simulink library "inp"  (R2021b)
settings: Solver=VariableStepAuto  StartTime=0.0  StopTime=10.0  RelTol=1e-3
undefined symbols (not defined in the file): C_TASK_5MS_S, FALSE, KINP_AcoreReadyToSlp_flg_ovrdflg, KINP_AcoreReadyToSlp_flg_ovrdval, KINP_AllowMovThd_OTA_enum_ovrdflg, KINP_AllowMovThd_OTA_enum_ovrdval, KINP_APSAngleTarget_Deg_ovrdflg, KINP_APSAngleTarget_Deg_ovrdval, KINP_APSDecReq_mps2_ovrdflg, KINP_APSDecReq_mps2_ovrdval, KINP_APSDecReqA_flg_ovrdflg, KINP_APSDecReqA_flg_ovrdval, KINP_APSDFLL_cm_ovrdflg, KINP_APSDFLL_cm_ovrdval, KINP_APSDFLR_cm_ovrdflg, KINP_APSDFLR_cm_ovrdval, KINP_APSDRLL_cm_ovrdflg, KINP_APSDRLL_cm_ovrdval, KINP_APSDRLR_cm_ovrdflg, KINP_APSDRLR_cm_ovrdval, KINP_APSExitCondition_enum_ovrdflg, KINP_APSExitCondition_enum_ovrdval, KINP_APSHWVer_enum_ovrdflg, KINP_APSHWVer_enum_ovrdval, KINP_APSProgressPCT_pct_ovrdflg, KINP_APSProgressPCT_pct_ovrdval, KINP_APSPwrReq_enum_ovrdflg, KINP_APSPwrReq_enum_ovrdval, KINP_APSReq_enum_ovrdflg, KINP_APSReq_enum_ovrdval, KINP_APSRQDisplay_enum_ovrdflg, KINP_APSRQDisplay_enum_ovrdval, KINP_APSRqEPASCtrl_flg_ovrdflg, KINP_APSRqEPASCtrl_flg_ovrdval, KINP_APSShiftPosnReq_enum_ovrdval, KINP_APSShiftPosnReq_enum_ovrflg, KINP_APSSpeedCMD_kph_ovrdval, KINP_APSSpeedCMD_kph_ovrflg, KINP_APSStaSystem_enum_ovrdflg, KINP_APSStaSystem_enum_ovrdval, KINP_APSSWVer_enum_ovrdflg, KINP_APSSWVer_enum_ovrdval, KINP_APSVMCReqA_flg_ovrdval, KINP_APSVMCReqA_flg_ovrflg, KINP_APSVRqEPASCtrl_flg_ovrdflg, KINP_APSVRqEPASCtrl_flg_ovrdval, KINP_AuxBattVolmV_mV_ovrdflg, KINP_AuxBattVolmV_mV_ovrdval, KINP_BTConnectSta_enum_ovrdflg, KINP_BTConnectSta_enum_ovrdval, KINP_CAASSta_enum_ovrdflg, KINP_CAASSta_enum_ovrdval, KINP_CAASVMCReqA_flg_ovrdval, KINP_CAASVMCReqA_flg_ovrflg, KINP_CAN1BusOff_flg_ovrdflg, KINP_CAN1BusOff_flg_ovrdval, KINP_CAN2BusOff_flg_ovrdflg, KINP_CAN2BusOff_flg_ovrdval, KINP_CAN3BusOff_flg_ovrdflg, KINP_CAN3BusOff_flg_ovrdval ... (+222)
libraries: FVT_lib x1035, hcu_lib x1
(part 14 of 33)

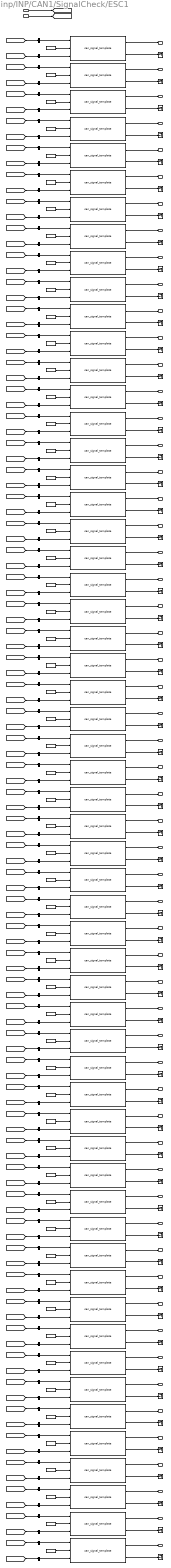
== system inp/INP/CAN1/SignalCheck/ESC1 ==
  BHAL_outputs : Inport
  inp_CanValid_bus : Inport  Port=2
  ABSActive : FVT_lib/inp/can_signal_template  SystemSampleTime=-1  VariantActivationTime=update diagram  Latency=0  AutoFrameSizeCalculation=off
      link override defval: Value=KINP_ABSActive_flg_defval
      link override ovrdflg: Value=KINP_ABSActive_flg_ovrdflg
      link override ovrdval: Value=KINP_ABSActive_flg_ovrdval
  ABSFailed : FVT_lib/inp/can_signal_template  SystemSampleTime=-1  VariantActivationTime=update diagram  Latency=0  AutoFrameSizeCalculation=off
      link override defval: Value=KINP_ABSFailed_flg_defval
      link override ovrdflg: Value=KINP_ABSFailed_flg_ovrdflg
      link override ovrdval: Value=KINP_ABSFailed_flg_ovrdval
  ABSWnlmpSta : FVT_lib/inp/can_signal_template  SystemSampleTime=-1  VariantActivationTime=update diagram  Latency=0  AutoFrameSizeCalculation=off
      link override defval: Value=KINP_ABSWnlmpSta_flg_defval
      link override ovrdflg: Value=KINP_ABSWnlmpSta_flg_ovrdflg
      link override ovrdval: Value=KINP_ABSWnlmpSta_flg_ovrdval
  AVHActive : FVT_lib/inp/can_signal_template  SystemSampleTime=-1  VariantActivationTime=update diagram  Latency=0  AutoFrameSizeCalculation=off
      link override defval: Value=KINP_AVHActive_flg_defval
      link override ovrdflg: Value=KINP_AVHActive_flg_ovrdflg
      link override ovrdval: Value=KINP_AVHActive_flg_ovrdval
  AVHFailed : FVT_lib/inp/can_signal_template  SystemSampleTime=-1  VariantActivationTime=update diagram  Latency=0  AutoFrameSizeCalculation=off
      link override defval: Value=KINP_AVHFailed_flg_defval
      link override ovrdflg: Value=KINP_AVHFailed_flg_ovrdflg
      link override ovrdval: Value=KINP_AVHFailed_flg_ovrdval
  AmberWnlmpSta : FVT_lib/inp/can_signal_template  SystemSampleTime=-1  VariantActivationTime=update diagram  Latency=0  AutoFrameSizeCalculation=off
      link override defval: Value=KINP_AmberWnlmpSta_flg_defval
      link override ovrdflg: Value=KINP_AmberWnlmpSta_flg_ovrdflg
      link override ovrdval: Value=KINP_AmberWnlmpSta_flg_ovrdval
  BTCSActive : FVT_lib/inp/can_signal_template  SystemSampleTime=-1  VariantActivationTime=update diagram  Latency=0  AutoFrameSizeCalculation=off
      link override defval: Value=KINP_BTCSActive_flg_defval
      link override ovrdflg: Value=KINP_BTCSActive_flg_ovrdflg
      link override ovrdval: Value=KINP_BTCSActive_flg_ovrdval
  EBDActive : FVT_lib/inp/can_signal_template  SystemSampleTime=-1  VariantActivationTime=update diagram  Latency=0  AutoFrameSizeCalculation=off
      link override defval: Value=KINP_EBDActive_flg_defval
      link override ovrdflg: Value=KINP_EBDActive_flg_ovrdflg
      link override ovrdval: Value=KINP_EBDActive_flg_ovrdval
  EBDFailed : FVT_lib/inp/can_signal_template  SystemSampleTime=-1  VariantActivationTime=update diagram  Latency=0  AutoFrameSizeCalculation=off
      link override defval: Value=KINP_EBDFailed_flg_defval
      link override ovrdflg: Value=KINP_EBDFailed_flg_ovrdflg
      link override ovrdval: Value=KINP_EBDFailed_flg_ovrdval
  ESC1CS : FVT_lib/inp/can_signal_template  SystemSampleTime=-1  VariantActivationTime=update diagram  Latency=0  AutoFrameSizeCalculation=off
      link override defval: Value=KINP_ESC1CS_enum_defval
      link override ovrdflg: Value=KINP_ESC1CS_enum_ovrdflg
      link override ovrdval: Value=KINP_ESC1CS_enum_ovrdval
  ESC1CSErr : FVT_lib/inp/can_signal_template  SystemSampleTime=-1  VariantActivationTime=update diagram  Latency=0  AutoFrameSizeCalculation=off
      link override defval: Value=KINP_ESC1CSErr_flg_defval
      link override ovrdflg: Value=KINP_ESC1CSErr_flg_ovrdflg
      link override ovrdval: Value=KINP_ESC1CSErr_flg_ovrdval
  ESC1RC : FVT_lib/inp/can_signal_template  SystemSampleTime=-1  VariantActivationTime=update diagram  Latency=0  AutoFrameSizeCalculation=off
      link override defval: Value=KINP_ESC1RC_enum_defval
      link override ovrdflg: Value=KINP_ESC1RC_enum_ovrdflg
      link override ovrdval: Value=KINP_ESC1RC_enum_ovrdval
  ESC1RCErr : FVT_lib/inp/can_signal_template  SystemSampleTime=-1  VariantActivationTime=update diagram  Latency=0  AutoFrameSizeCalculation=off
      link override defval: Value=KINP_ESC1RCErr_flg_defval
      link override ovrdflg: Value=KINP_ESC1RCErr_flg_ovrdflg
      link override ovrdval: Value=KINP_ESC1RCErr_flg_ovrdval
  ESCActive : FVT_lib/inp/can_signal_template  SystemSampleTime=-1  VariantActivationTime=update diagram  Latency=0  AutoFrameSizeCalculation=off
      link override defval: Value=KINP_ESCActive_flg_defval
      link override ovrdflg: Value=KINP_ESCActive_flg_ovrdflg
      link override ovrdval: Value=KINP_ESCActive_flg_ovrdval
  ESCBeepReq : FVT_lib/inp/can_signal_template  SystemSampleTime=-1  VariantActivationTime=update diagram  Latency=0  AutoFrameSizeCalculation=off
      link override defval: Value=KINP_ESCBeepReq_flg_defval
      link override ovrdflg: Value=KINP_ESCBeepReq_flg_ovrdflg
      link override ovrdval: Value=KINP_ESCBeepReq_flg_ovrdval
  ESCFailed : FVT_lib/inp/can_signal_template  SystemSampleTime=-1  VariantActivationTime=update diagram  Latency=0  AutoFrameSizeCalculation=off
      link override defval: Value=KINP_ESCFailed_flg_defval
      link override ovrdflg: Value=KINP_ESCFailed_flg_ovrdflg
      link override ovrdval: Value=KINP_ESCFailed_flg_ovrdval
  ESCOFFStatus : FVT_lib/inp/can_signal_template  SystemSampleTime=-1  VariantActivationTime=update diagram  Latency=0  AutoFrameSizeCalculation=off
      link override defval: Value=KINP_ESCOFFStatus_enum_defval
      link override ovrdflg: Value=KINP_ESCOFFStatus_enum_ovrdflg
      link override ovrdval: Value=KINP_ESCOFFStatus_enum_ovrdval
  ESCOfflmpSta : FVT_lib/inp/can_signal_template  SystemSampleTime=-1  VariantActivationTime=update diagram  Latency=0  AutoFrameSizeCalculation=off
      link override defval: Value=KINP_ESCOfflmpSta_flg_defval
      link override ovrdflg: Value=KINP_ESCOfflmpSta_flg_ovrdflg
      link override ovrdval: Value=KINP_ESCOfflmpSta_flg_ovrdval
  ESCWnlmpSta : FVT_lib/inp/can_signal_template  SystemSampleTime=-1  VariantActivationTime=update diagram  Latency=0  AutoFrameSizeCalculation=off
      link override defval: Value=KINP_ESCWnlmpSta_enum_defval
      link override ovrdflg: Value=KINP_ESCWnlmpSta_enum_ovrdflg
      link override ovrdval: Value=KINP_ESCWnlmpSta_enum_ovrdval
  ESSActive : FVT_lib/inp/can_signal_template  SystemSampleTime=-1  VariantActivationTime=update diagram  Latency=0  AutoFrameSizeCalculation=off
      link override defval: Value=KINP_ESSActive_flg_defval
      link override ovrdflg: Value=KINP_ESSActive_flg_ovrdflg
      link override ovrdval: Value=KINP_ESSActive_flg_ovrdval
  FrPTCSActive : FVT_lib/inp/can_signal_template  SystemSampleTime=-1  VariantActivationTime=update diagram  Latency=0  AutoFrameSizeCalculation=off
      link override defval: Value=KINP_FrPTCSActive_flg_defval
      link override ovrdflg: Value=KINP_FrPTCSActive_flg_ovrdflg
      link override ovrdval: Value=KINP_FrPTCSActive_flg_ovrdval
  FrntAxlTrqReqDrv : FVT_lib/inp/can_signal_template  SystemSampleTime=-1  VariantActivationTime=update diagram  Latency=0  AutoFrameSizeCalculation=off
      link override defval: Value=KINP_FrntAxlTrqReqDrv_Nm_defval
      link override ovrdflg: Value=KINP_FrntAxlTrqReqDrv_Nm_ovrdflg
      link override ovrdval: Value=KINP_FrntAxlTrqReqDrv_Nm_ovrdval
  GRADE : FVT_lib/inp/can_signal_template  SystemSampleTime=-1  VariantActivationTime=update diagram  Latency=0  AutoFrameSizeCalculation=off
      link override defval: Value=KINP_GRADE_Deg_defval
      link override ovrdflg: Value=KINP_GRADE_Deg_ovrdflg
      link override ovrdval: Value=KINP_GRADE_Deg_ovrdval
  HBBActive : FVT_lib/inp/can_signal_template  SystemSampleTime=-1  VariantActivationTime=update diagram  Latency=0  AutoFrameSizeCalculation=off
      link override defval: Value=KINP_HBBActive_flg_defval
      link override ovrdflg: Value=KINP_HBBActive_flg_ovrdflg
      link override ovrdval: Value=KINP_HBBActive_flg_ovrdval
  HBBFailed : FVT_lib/inp/can_signal_template  SystemSampleTime=-1  VariantActivationTime=update diagram  Latency=0  AutoFrameSizeCalculation=off
      link override defval: Value=KINP_HBBFailed_flg_defval
      link override ovrdflg: Value=KINP_HBBFailed_flg_ovrdflg
      link override ovrdval: Value=KINP_HBBFailed_flg_ovrdval
  HDDActive : FVT_lib/inp/can_signal_template  SystemSampleTime=-1  VariantActivationTime=update diagram  Latency=0  AutoFrameSizeCalculation=off
      link override defval: Value=KINP_HDDActive_flg_defval
      link override ovrdflg: Value=KINP_HDDActive_flg_ovrdflg
      link override ovrdval: Value=KINP_HDDActive_flg_ovrdval
  HDDFailed : FVT_lib/inp/can_signal_template  SystemSampleTime=-1  VariantActivationTime=update diagram  Latency=0  AutoFrameSizeCalculation=off
      link override defval: Value=KINP_HDDFailed_flg_defval
      link override ovrdflg: Value=KINP_HDDFailed_flg_ovrdflg
      link override ovrdval: Value=KINP_HDDFailed_flg_ovrdval
  HSAActive : FVT_lib/inp/can_signal_template  SystemSampleTime=-1  VariantActivationTime=update diagram  Latency=0  AutoFrameSizeCalculation=off
      link override defval: Value=KINP_HSAActive_flg_defval
      link override ovrdflg: Value=KINP_HSAActive_flg_ovrdflg
      link override ovrdval: Value=KINP_HSAActive_flg_ovrdval
  HSAFailed : FVT_lib/inp/can_signal_template  SystemSampleTime=-1  VariantActivationTime=update diagram  Latency=0  AutoFrameSizeCalculation=off
      link override defval: Value=KINP_HSAFailed_flg_defval
      link override ovrdflg: Value=KINP_HSAFailed_flg_ovrdflg
      link override ovrdval: Value=KINP_HSAFailed_flg_ovrdval
  LFPulseCount : FVT_lib/inp/can_signal_template  SystemSampleTime=-1  VariantActivationTime=update diagram  Latency=0  AutoFrameSizeCalculation=off
      link override defval: Value=KINP_LFPulseCount_enum_defval
      link override ovrdflg: Value=KINP_LFPulseCount_enum_ovrdflg
      link override ovrdval: Value=KINP_LFPulseCount_enum_ovrdval
  LFPulseCountV : FVT_lib/inp/can_signal_template  SystemSampleTime=-1  VariantActivationTime=update diagram  Latency=0  AutoFrameSizeCalculation=off
      link override defval: Value=KINP_LFPulseCountV_flg_defval
      link override ovrdflg: Value=KINP_LFPulseCountV_flg_ovrdflg
      link override ovrdval: Value=KINP_LFPulseCountV_flg_ovrdval
  LFRawWhlSpeed : FVT_lib/inp/can_signal_template  SystemSampleTime=-1  VariantActivationTime=update diagram  Latency=0  AutoFrameSizeCalculation=off
      link override defval: Value=KINP_LFRawWhlSpeed_kph_defval
      link override ovrdflg: Value=KINP_LFRawWhlSpeed_kph_ovrdflg
      link override ovrdval: Value=KINP_LFRawWhlSpeed_kph_ovrdval
  LFRawWhlSpeedV : FVT_lib/inp/can_signal_template  SystemSampleTime=-1  VariantActivationTime=update diagram  Latency=0  AutoFrameSizeCalculation=off
      link override defval: Value=KINP_LFRawWhlSpeedV_flg_defval
      link override ovrdflg: Value=KINP_LFRawWhlSpeedV_flg_ovrdflg
      link override ovrdval: Value=KINP_LFRawWhlSpeedV_flg_ovrdval
  LFWhlRotDir : FVT_lib/inp/can_signal_template  SystemSampleTime=-1  VariantActivationTime=update diagram  Latency=0  AutoFrameSizeCalculation=off
      link override defval: Value=KINP_LFWhlRotDir_enum_defval
      link override ovrdflg: Value=KINP_LFWhlRotDir_enum_ovrdflg
      link override ovrdval: Value=KINP_LFWhlRotDir_enum_ovrdval
  LRPulseCount : FVT_lib/inp/can_signal_template  SystemSampleTime=-1  VariantActivationTime=update diagram  Latency=0  AutoFrameSizeCalculation=off
      link override defval: Value=KINP_LRPulseCount_enum_defval
      link override ovrdflg: Value=KINP_LRPulseCount_enum_ovrdflg
      link override ovrdval: Value=KINP_LRPulseCount_enum_ovrdval
  LRPulseCountV : FVT_lib/inp/can_signal_template  SystemSampleTime=-1  VariantActivationTime=update diagram  Latency=0  AutoFrameSizeCalculation=off
      link override defval: Value=KINP_LRPulseCountV_flg_defval
      link override ovrdflg: Value=KINP_LRPulseCountV_flg_ovrdflg
      link override ovrdval: Value=KINP_LRPulseCountV_flg_ovrdval
  LRRawWhlSpeed : FVT_lib/inp/can_signal_template  SystemSampleTime=-1  VariantActivationTime=update diagram  Latency=0  AutoFrameSizeCalculation=off
      link override defval: Value=KINP_LRRawWhlSpeed_kph_defval
      link override ovrdflg: Value=KINP_LRRawWhlSpeed_kph_ovrdflg
      link override ovrdval: Value=KINP_LRRawWhlSpeed_kph_ovrdval
  LRRawWhlSpeedV : FVT_lib/inp/can_signal_template  SystemSampleTime=-1  VariantActivationTime=update diagram  Latency=0  AutoFrameSizeCalculation=off
      link override defval: Value=KINP_LRRawWhlSpeedV_flg_defval
      link override ovrdflg: Value=KINP_LRRawWhlSpeedV_flg_ovrdflg
      link override ovrdval: Value=KINP_LRRawWhlSpeedV_flg_ovrdval
  LRWhlRotDir : FVT_lib/inp/can_signal_template  SystemSampleTime=-1  VariantActivationTime=update diagram  Latency=0  AutoFrameSizeCalculation=off
      link override defval: Value=KINP_LRWhlRotDir_enum_defval
      link override ovrdflg: Value=KINP_LRWhlRotDir_enum_ovrdflg
      link override ovrdval: Value=KINP_LRWhlRotDir_enum_ovrdval
  PBAActive : FVT_lib/inp/can_signal_template  SystemSampleTime=-1  VariantActivationTime=update diagram  Latency=0  AutoFrameSizeCalculation=off
      link override defval: Value=KINP_PBAActive_flg_defval
      link override ovrdflg: Value=KINP_PBAActive_flg_ovrdflg
      link override ovrdval: Value=KINP_PBAActive_flg_ovrdval
  PBAFailed : FVT_lib/inp/can_signal_template  SystemSampleTime=-1  VariantActivationTime=update diagram  Latency=0  AutoFrameSizeCalculation=off
      link override defval: Value=KINP_PBAFailed_flg_defval
      link override ovrdflg: Value=KINP_PBAFailed_flg_ovrdflg
      link override ovrdval: Value=KINP_PBAFailed_flg_ovrdval
  RFPulseCount : FVT_lib/inp/can_signal_template  SystemSampleTime=-1  VariantActivationTime=update diagram  Latency=0  AutoFrameSizeCalculation=off
      link override defval: Value=KINP_RFPulseCount_enum_defval
      link override ovrdflg: Value=KINP_RFPulseCount_enum_ovrdflg
      link override ovrdval: Value=KINP_RFPulseCount_enum_ovrdval
  RFPulseCountV : FVT_lib/inp/can_signal_template  SystemSampleTime=-1  VariantActivationTime=update diagram  Latency=0  AutoFrameSizeCalculation=off
      link override defval: Value=KINP_RFPulseCountV_flg_defval
      link override ovrdflg: Value=KINP_RFPulseCountV_flg_ovrdflg
      link override ovrdval: Value=KINP_RFPulseCountV_flg_ovrdval
  RFRawWhlSpeed : FVT_lib/inp/can_signal_template  SystemSampleTime=-1  VariantActivationTime=update diagram  Latency=0  AutoFrameSizeCalculation=off
      link override defval: Value=KINP_RFRawWhlSpeed_kph_defval
      link override ovrdflg: Value=KINP_RFRawWhlSpeed_kph_ovrdflg
      link override ovrdval: Value=KINP_RFRawWhlSpeed_kph_ovrdval
  RFRawWhlSpeedV : FVT_lib/inp/can_signal_template  SystemSampleTime=-1  VariantActivationTime=update diagram  Latency=0  AutoFrameSizeCalculation=off
      link override defval: Value=KINP_RFRawWhlSpeedV_flg_defval
      link override ovrdflg: Value=KINP_RFRawWhlSpeedV_flg_ovrdflg
      link override ovrdval: Value=KINP_RFRawWhlSpeedV_flg_ovrdval
  RFWhlRotDir : FVT_lib/inp/can_signal_template  SystemSampleTime=-1  VariantActivationTime=update diagram  Latency=0  AutoFrameSizeCalculation=off
      link override defval: Value=KINP_RFWhlRotDir_enum_defval
      link override ovrdflg: Value=KINP_RFWhlRotDir_enum_ovrdflg
      link override ovrdval: Value=KINP_RFWhlRotDir_enum_ovrdval
  RRPulseCount : FVT_lib/inp/can_signal_template  SystemSampleTime=-1  VariantActivationTime=update diagram  Latency=0  AutoFrameSizeCalculation=off
      link override defval: Value=KINP_RRPulseCount_enum_defval
      link override ovrdflg: Value=KINP_RRPulseCount_enum_ovrdflg
      link override ovrdval: Value=KINP_RRPulseCount_enum_ovrdval
  RRPulseCountV : FVT_lib/inp/can_signal_template  SystemSampleTime=-1  VariantActivationTime=update diagram  Latency=0  AutoFrameSizeCalculation=off
      link override defval: Value=KINP_RRPulseCountV_flg_defval
      link override ovrdflg: Value=KINP_RRPulseCountV_flg_ovrdflg
      link override ovrdval: Value=KINP_RRPulseCountV_flg_ovrdval
  RRRawWhlSpeed : FVT_lib/inp/can_signal_template  SystemSampleTime=-1  VariantActivationTime=update diagram  Latency=0  AutoFrameSizeCalculation=off
      link override defval: Value=KINP_RRRawWhlSpeed_kph_defval
      link override ovrdflg: Value=KINP_RRRawWhlSpeed_kph_ovrdflg
      link override ovrdval: Value=KINP_RRRawWhlSpeed_kph_ovrdval
  RRRawWhlSpeedV : FVT_lib/inp/can_signal_template  SystemSampleTime=-1  VariantActivationTime=update diagram  Latency=0  AutoFrameSizeCalculation=off
      link override defval: Value=KINP_RRRawWhlSpeedV_flg_defval
      link override ovrdflg: Value=KINP_RRRawWhlSpeedV_flg_ovrdflg
      link override ovrdval: Value=KINP_RRRawWhlSpeedV_flg_ovrdval
  RRWhlRotDir : FVT_lib/inp/can_signal_template  SystemSampleTime=-1  VariantActivationTime=update diagram  Latency=0  AutoFrameSizeCalculation=off
      link override defval: Value=KINP_RRWhlRotDir_enum_defval
      link override ovrdflg: Value=KINP_RRWhlRotDir_enum_ovrdflg
      link override ovrdval: Value=KINP_RRWhlRotDir_enum_ovrdval
  RearAxlTrqReqDrv : FVT_lib/inp/can_signal_template  SystemSampleTime=-1  VariantActivationTime=update diagram  Latency=0  AutoFrameSizeCalculation=off
      link override defval: Value=KINP_RearAxlTrqReqDrv_Nm_defval
      link override ovrdflg: Value=KINP_RearAxlTrqReqDrv_Nm_ovrdflg
      link override ovrdval: Value=KINP_RearAxlTrqReqDrv_Nm_ovrdval
  RedWnlmpSta : FVT_lib/inp/can_signal_template  SystemSampleTime=-1  VariantActivationTime=update diagram  Latency=0  AutoFrameSizeCalculation=off
      link override defval: Value=KINP_RedWnlmpSta_flg_defval
      link override ovrdflg: Value=KINP_RedWnlmpSta_flg_ovrdflg
      link override ovrdval: Value=KINP_RedWnlmpSta_flg_ovrdval
  RrPTCSActive : FVT_lib/inp/can_signal_template  SystemSampleTime=-1  VariantActivationTime=update diagram  Latency=0  AutoFrameSizeCalculation=off
      link override defval: Value=KINP_RrPTCSActive_flg_defval
      link override ovrdflg: Value=KINP_RrPTCSActive_flg_ovrdflg
      link override ovrdval: Value=KINP_RrPTCSActive_flg_ovrdval
  TCSActive : FVT_lib/inp/can_signal_template  SystemSampleTime=-1  VariantActivationTime=update diagram  Latency=0  AutoFrameSizeCalculation=off
      link override defval: Value=KINP_TCSActive_flg_defval
      link override ovrdflg: Value=KINP_TCSActive_flg_ovrdflg
      link override ovrdval: Value=KINP_TCSActive_flg_ovrdval
  TCSFailed : FVT_lib/inp/can_signal_template  SystemSampleTime=-1  VariantActivationTime=update diagram  Latency=0  AutoFrameSizeCalculation=off
      link override defval: Value=KINP_TCSFailed_flg_defval
      link override ovrdflg: Value=KINP_TCSFailed_flg_ovrdflg
      link override ovrdval: Value=KINP_TCSFailed_flg_ovrdval
  Terminator_{1..57} (57 alike) : Terminator
  True_VHAL_ABSActive_flg : Constant  Value=TRUE  OutDataTypeStr=boolean
  True_VHAL_ABSFailed_flg : Constant  Value=TRUE  OutDataTypeStr=boolean
  True_VHAL_ABSWnlmpSta_flg : Constant  Value=TRUE  OutDataTypeStr=boolean
  True_VHAL_AVHActive_flg : Constant  Value=TRUE  OutDataTypeStr=boolean
  True_VHAL_AVHFailed_flg : Constant  Value=TRUE  OutDataTypeStr=boolean
  True_VHAL_AmberWnlmpSta_flg : Constant  Value=TRUE  OutDataTypeStr=boolean
  True_VHAL_BTCSActive_flg : Constant  Value=TRUE  OutDataTypeStr=boolean
  True_VHAL_EBDActive_flg : Constant  Value=TRUE  OutDataTypeStr=boolean
  True_VHAL_EBDFailed_flg : Constant  Value=TRUE  OutDataTypeStr=boolean
  True_VHAL_ESC1CSErr_flg : Constant  Value=TRUE  OutDataTypeStr=boolean
  True_VHAL_ESC1CS_enum : Constant  Value=TRUE  OutDataTypeStr=boolean
  True_VHAL_ESC1RCErr_flg : Constant  Value=TRUE  OutDataTypeStr=boolean
  True_VHAL_ESC1RC_enum : Constant  Value=TRUE  OutDataTypeStr=boolean
  True_VHAL_ESCActive_flg : Constant  Value=TRUE  OutDataTypeStr=boolean
  True_VHAL_ESCBeepReq_flg : Constant  Value=TRUE  OutDataTypeStr=boolean
  True_VHAL_ESCFailed_flg : Constant  Value=TRUE  OutDataTypeStr=boolean
  True_VHAL_ESCOFFStatus_enum : Constant  Value=TRUE  OutDataTypeStr=boolean
  True_VHAL_ESCOfflmpSta_flg : Constant  Value=TRUE  OutDataTypeStr=boolean
  True_VHAL_ESCWnlmpSta_enum : Constant  Value=TRUE  OutDataTypeStr=boolean
  True_VHAL_ESSActive_flg : Constant  Value=TRUE  OutDataTypeStr=boolean
  True_VHAL_FrPTCSActive_flg : Constant  Value=TRUE  OutDataTypeStr=boolean
  True_VHAL_FrntAxlTrqReqDrv_Nm : Constant  Value=TRUE  OutDataTypeStr=boolean
  True_VHAL_GRADE_Deg : Constant  Value=TRUE  OutDataTypeStr=boolean
  True_VHAL_HBBActive_flg : Constant  Value=TRUE  OutDataTypeStr=boolean
  True_VHAL_HBBFailed_flg : Constant  Value=TRUE  OutDataTypeStr=boolean
  True_VHAL_HDDActive_flg : Constant  Value=TRUE  OutDataTypeStr=boolean
  True_VHAL_HDDFailed_flg : Constant  Value=TRUE  OutDataTypeStr=boolean
  True_VHAL_HSAActive_flg : Constant  Value=TRUE  OutDataTypeStr=boolean
  True_VHAL_HSAFailed_flg : Constant  Value=TRUE  OutDataTypeStr=boolean
  True_VHAL_LFPulseCountV_flg : Constant  Value=TRUE  OutDataTypeStr=boolean
  True_VHAL_LFPulseCount_enum : Constant  Value=TRUE  OutDataTypeStr=boolean
  True_VHAL_LFRawWhlSpeedV_flg : Constant  Value=TRUE  OutDataTypeStr=boolean
  True_VHAL_LFRawWhlSpeed_kph : Constant  Value=TRUE  OutDataTypeStr=boolean
  True_VHAL_LFWhlRotDir_enum : Constant  Value=TRUE  OutDataTypeStr=boolean
  True_VHAL_LRPulseCountV_flg : Constant  Value=TRUE  OutDataTypeStr=boolean
  True_VHAL_LRPulseCount_enum : Constant  Value=TRUE  OutDataTypeStr=boolean
  True_VHAL_LRRawWhlSpeedV_flg : Constant  Value=TRUE  OutDataTypeStr=boolean
  True_VHAL_LRRawWhlSpeed_kph : Constant  Value=TRUE  OutDataTypeStr=boolean
  True_VHAL_LRWhlRotDir_enum : Constant  Value=TRUE  OutDataTypeStr=boolean
  True_VHAL_PBAActive_flg : Constant  Value=TRUE  OutDataTypeStr=boolean
  True_VHAL_PBAFailed_flg : Constant  Value=TRUE  OutDataTypeStr=boolean
  True_VHAL_RFPulseCountV_flg : Constant  Value=TRUE  OutDataTypeStr=boolean
  True_VHAL_RFPulseCount_enum : Constant  Value=TRUE  OutDataTypeStr=boolean
  True_VHAL_RFRawWhlSpeedV_flg : Constant  Value=TRUE  OutDataTypeStr=boolean
  True_VHAL_RFRawWhlSpeed_kph : Constant  Value=TRUE  OutDataTypeStr=boolean
  True_VHAL_RFWhlRotDir_enum : Constant  Value=TRUE  OutDataTypeStr=boolean
  True_VHAL_RRPulseCountV_flg : Constant  Value=TRUE  OutDataTypeStr=boolean
  True_VHAL_RRPulseCount_enum : Constant  Value=TRUE  OutDataTypeStr=boolean
  True_VHAL_RRRawWhlSpeedV_flg : Constant  Value=TRUE  OutDataTypeStr=boolean
  True_VHAL_RRRawWhlSpeed_kph : Constant  Value=TRUE  OutDataTypeStr=boolean
  True_VHAL_RRWhlRotDir_enum : Constant  Value=TRUE  OutDataTypeStr=boolean
  True_VHAL_RearAxlTrqReqDrv_Nm : Constant  Value=TRUE  OutDataTypeStr=boolean
  True_VHAL_RedWnlmpSta_flg : Constant  Value=TRUE  OutDataTypeStr=boolean
  True_VHAL_RrPTCSActive_flg : Constant  Value=TRUE  OutDataTypeStr=boolean
  True_VHAL_TCSActive_flg : Constant  Value=TRUE  OutDataTypeStr=boolean
  True_VHAL_TCSFailed_flg : Constant  Value=TRUE  OutDataTypeStr=boolean
  True_VHAL_VehSpeed_kph : Constant  Value=TRUE  OutDataTypeStr=boolean
  VehSpeed : FVT_lib/inp/can_signal_template  SystemSampleTime=-1  VariantActivationTime=update diagram  Latency=0  AutoFrameSizeCalculation=off
      link override defval: Value=KINP_VehSpeed_kph_defval
      link override ovrdflg: Value=KINP_VehSpeed_kph_ovrdflg
      link override ovrdval: Value=KINP_VehSpeed_kph_ovrdval
  slr1_{1..57} (57 alike) : BusSelector  OutputSignals=VINP_CANMsgValidESC1_flg
  slr_VHAL_ABSActive_flg : BusSelector  OutputSignals=VHAL_ABSActive_flg
  slr_VHAL_ABSFailed_flg : BusSelector  OutputSignals=VHAL_ABSFailed_flg
  slr_VHAL_ABSWnlmpSta_flg : BusSelector  OutputSignals=VHAL_ABSWnlmpSta_flg
  slr_VHAL_AVHActive_flg : BusSelector  OutputSignals=VHAL_AVHActive_flg
  slr_VHAL_AVHFailed_flg : BusSelector  OutputSignals=VHAL_AVHFailed_flg
  slr_VHAL_AmberWnlmpSta_flg : BusSelector  OutputSignals=VHAL_AmberWnlmpSta_flg
  slr_VHAL_BTCSActive_flg : BusSelector  OutputSignals=VHAL_BTCSActive_flg
  slr_VHAL_EBDActive_flg : BusSelector  OutputSignals=VHAL_EBDActive_flg
  slr_VHAL_EBDFailed_flg : BusSelector  OutputSignals=VHAL_EBDFailed_flg
  slr_VHAL_ESC1CSErr_flg : BusSelector  OutputSignals=VHAL_ESC1CSErr_flg
  slr_VHAL_ESC1CS_enum : BusSelector  OutputSignals=VHAL_ESC1CS_enum
  slr_VHAL_ESC1RCErr_flg : BusSelector  OutputSignals=VHAL_ESC1RCErr_flg
  slr_VHAL_ESC1RC_enum : BusSelector  OutputSignals=VHAL_ESC1RC_enum
  slr_VHAL_ESCActive_flg : BusSelector  OutputSignals=VHAL_ESCActive_flg
  slr_VHAL_ESCBeepReq_flg : BusSelector  OutputSignals=VHAL_ESCBeepReq_flg
  slr_VHAL_ESCFailed_flg : BusSelector  OutputSignals=VHAL_ESCFailed_flg
  slr_VHAL_ESCOFFStatus_enum : BusSelector  OutputSignals=VHAL_ESCOFFStatus_enum
  slr_VHAL_ESCOfflmpSta_flg : BusSelector  OutputSignals=VHAL_ESCOfflmpSta_flg
  slr_VHAL_ESCWnlmpSta_enum : BusSelector  OutputSignals=VHAL_ESCWnlmpSta_enum
  slr_VHAL_ESSActive_flg : BusSelector  OutputSignals=VHAL_ESSActive_flg
  slr_VHAL_FrPTCSActive_flg : BusSelector  OutputSignals=VHAL_FrPTCSActive_flg
  slr_VHAL_FrntAxlTrqReqDrv_Nm : BusSelector  OutputSignals=VHAL_FrntAxlTrqReqDrv_Nm
  slr_VHAL_GRADE_Deg : BusSelector  OutputSignals=VHAL_GRADE_Deg
  slr_VHAL_HBBActive_flg : BusSelector  OutputSignals=VHAL_HBBActive_flg
  slr_VHAL_HBBFailed_flg : BusSelector  OutputSignals=VHAL_HBBFailed_flg
  slr_VHAL_HDDActive_flg : BusSelector  OutputSignals=VHAL_HDDActive_flg
  slr_VHAL_HDDFailed_flg : BusSelector  OutputSignals=VHAL_HDDFailed_flg
  slr_VHAL_HSAActive_flg : BusSelector  OutputSignals=VHAL_HSAActive_flg
  slr_VHAL_HSAFailed_flg : BusSelector  OutputSignals=VHAL_HSAFailed_flg
  slr_VHAL_LFPulseCountV_flg : BusSelector  OutputSignals=VHAL_LFPulseCountV_flg
  slr_VHAL_LFPulseCount_enum : BusSelector  OutputSignals=VHAL_LFPulseCount_enum
  slr_VHAL_LFRawWhlSpeedV_flg : BusSelector  OutputSignals=VHAL_LFRawWhlSpeedV_flg
  slr_VHAL_LFRawWhlSpeed_kph : BusSelector  OutputSignals=VHAL_LFRawWhlSpeed_kph
  slr_VHAL_LFWhlRotDir_enum : BusSelector  OutputSignals=VHAL_LFWhlRotDir_enum
  slr_VHAL_LRPulseCountV_flg : BusSelector  OutputSignals=VHAL_LRPulseCountV_flg
  slr_VHAL_LRPulseCount_enum : BusSelector  OutputSignals=VHAL_LRPulseCount_enum
  slr_VHAL_LRRawWhlSpeedV_flg : BusSelector  OutputSignals=VHAL_LRRawWhlSpeedV_flg
  slr_VHAL_LRRawWhlSpeed_kph : BusSelector  OutputSignals=VHAL_LRRawWhlSpeed_kph
  slr_VHAL_LRWhlRotDir_enum : BusSelector  OutputSignals=VHAL_LRWhlRotDir_enum
  slr_VHAL_PBAActive_flg : BusSelector  OutputSignals=VHAL_PBAActive_flg
  slr_VHAL_PBAFailed_flg : BusSelector  OutputSignals=VHAL_PBAFailed_flg
  slr_VHAL_RFPulseCountV_flg : BusSelector  OutputSignals=VHAL_RFPulseCountV_flg
  slr_VHAL_RFPulseCount_enum : BusSelector  OutputSignals=VHAL_RFPulseCount_enum
  slr_VHAL_RFRawWhlSpeedV_flg : BusSelector  OutputSignals=VHAL_RFRawWhlSpeedV_flg
  slr_VHAL_RFRawWhlSpeed_kph : BusSelector  OutputSignals=VHAL_RFRawWhlSpeed_kph
  slr_VHAL_RFWhlRotDir_enum : BusSelector  OutputSignals=VHAL_RFWhlRotDir_enum
  slr_VHAL_RRPulseCountV_flg : BusSelector  OutputSignals=VHAL_RRPulseCountV_flg
  slr_VHAL_RRPulseCount_enum : BusSelector  OutputSignals=VHAL_RRPulseCount_enum
  slr_VHAL_RRRawWhlSpeedV_flg : BusSelector  OutputSignals=VHAL_RRRawWhlSpeedV_flg
  slr_VHAL_RRRawWhlSpeed_kph : BusSelector  OutputSignals=VHAL_RRRawWhlSpeed_kph
  slr_VHAL_RRWhlRotDir_enum : BusSelector  OutputSignals=VHAL_RRWhlRotDir_enum
  slr_VHAL_RearAxlTrqReqDrv_Nm : BusSelector  OutputSignals=VHAL_RearAxlTrqReqDrv_Nm
  slr_VHAL_RedWnlmpSta_flg : BusSelector  OutputSignals=VHAL_RedWnlmpSta_flg
  slr_VHAL_RrPTCSActive_flg : BusSelector  OutputSignals=VHAL_RrPTCSActive_flg
  slr_VHAL_TCSActive_flg : BusSelector  OutputSignals=VHAL_TCSActive_flg
  slr_VHAL_TCSFailed_flg : BusSelector  OutputSignals=VHAL_TCSFailed_flg
  slr_VHAL_VehSpeed_kph : BusSelector  OutputSignals=VHAL_VehSpeed_kph
  VINP_ESC1CSErr_flg : Outport
  VINP_ESC1RCErr_flg : Outport  Port=2
  VINP_ABSActive_flg : Outport  Port=3
  VINP_ABSFailed_flg : Outport  Port=4
  VINP_ABSWnlmpSta_flg : Outport  Port=5
  VINP_AVHActive_flg : Outport  Port=6
  VINP_AVHFailed_flg : Outport  Port=7
  VINP_AmberWnlmpSta_flg : Outport  Port=8
  VINP_BTCSActive_flg : Outport  Port=9
  VINP_EBDActive_flg : Outport  Port=10
  VINP_EBDFailed_flg : Outport  Port=11
  VINP_ESC1CS_enum : Outport  Port=12
  VINP_ESC1RC_enum : Outport  Port=13
  VINP_ESCActive_flg : Outport  Port=14
  VINP_ESCBeepReq_flg : Outport  Port=15
  VINP_ESCFailed_flg : Outport  Port=16
  VINP_ESCOFFStatus_enum : Outport  Port=17
  VINP_ESCOfflmpSta_flg : Outport  Port=18
  VINP_ESCWnlmpSta_enum : Outport  Port=19
  VINP_ESSActive_flg : Outport  Port=20
  VINP_FrPTCSActive_flg : Outport  Port=21
  VINP_FrntAxlTrqReqDrv_Nm : Outport  Port=22
  VINP_GRADE_Deg : Outport  Port=23
  VINP_HBBActive_flg : Outport  Port=24
  VINP_HBBFailed_flg : Outport  Port=25
  VINP_HDDActive_flg : Outport  Port=26
  VINP_HDDFailed_flg : Outport  Port=27
  VINP_HSAActive_flg : Outport  Port=28
  VINP_HSAFailed_flg : Outport  Port=29
  VINP_LFPulseCount_enum : Outport  Port=30
  VINP_LFPulseCountV_flg : Outport  Port=31
  VINP_LFRawWhlSpeed_kph : Outport  Port=32
  VINP_LFRawWhlSpeedV_flg : Outport  Port=33
  VINP_LFWhlRotDir_enum : Outport  Port=34
  VINP_LRPulseCount_enum : Outport  Port=35
  VINP_LRPulseCountV_flg : Outport  Port=36
  VINP_LRRawWhlSpeed_kph : Outport  Port=37
  VINP_LRRawWhlSpeedV_flg : Outport  Port=38
  VINP_LRWhlRotDir_enum : Outport  Port=39
  VINP_PBAActive_flg : Outport  Port=40
  VINP_PBAFailed_flg : Outport  Port=41
  VINP_RFPulseCount_enum : Outport  Port=42
  VINP_RFPulseCountV_flg : Outport  Port=43
  VINP_RFRawWhlSpeed_kph : Outport  Port=44
  VINP_RFRawWhlSpeedV_flg : Outport  Port=45
  VINP_RFWhlRotDir_enum : Outport  Port=46
  VINP_RRPulseCount_enum : Outport  Port=47
  VINP_RRPulseCountV_flg : Outport  Port=48
  VINP_RRRawWhlSpeed_kph : Outport  Port=49
  VINP_RRRawWhlSpeedV_flg : Outport  Port=50
  VINP_RRWhlRotDir_enum : Outport  Port=51
  VINP_RearAxlTrqReqDrv_Nm : Outport  Port=52
  VINP_RedWnlmpSta_flg : Outport  Port=53
  VINP_RrPTCSActive_flg : Outport  Port=54
  VINP_TCSActive_flg : Outport  Port=55
  VINP_TCSFailed_flg : Outport  Port=56
  VINP_VehSpeed_kph : Outport  Port=57
  wires:
  BHAL_outputs/1 -> [BHAL_outputs]
  inp_CanValid_bus/1 -> [inp_CanValid_bus]
  [BHAL_outputs] -> slr_VHAL_ESC1CSErr_flg/1
  slr_VHAL_ESC1CSErr_flg/1 -> ESC1CSErr/1  "<VHAL_ESC1CSErr_flg>"
  True_VHAL_ESC1CSErr_flg/1 -> ESC1CSErr/2
  [inp_CanValid_bus] -> slr1_1/1
  slr1_1/1 -> ESC1CSErr/3  "<VINP_CANMsgValidESC1_flg>"
  ESC1CSErr/1 -> VINP_ESC1CSErr_flg/1  "VINP_ESC1CSErr_flg"
  ESC1CSErr/2 -> Terminator_1/1
  [BHAL_outputs] -> slr_VHAL_ESC1RCErr_flg/1
  slr_VHAL_ESC1RCErr_flg/1 -> ESC1RCErr/1  "<VHAL_ESC1RCErr_flg>"
  True_VHAL_ESC1RCErr_flg/1 -> ESC1RCErr/2
  [inp_CanValid_bus] -> slr1_2/1
  slr1_2/1 -> ESC1RCErr/3  "<VINP_CANMsgValidESC1_flg>"
  ESC1RCErr/1 -> VINP_ESC1RCErr_flg/1  "VINP_ESC1RCErr_flg"
  ESC1RCErr/2 -> Terminator_2/1
  [BHAL_outputs] -> slr_VHAL_ABSActive_flg/1
  slr_VHAL_ABSActive_flg/1 -> ABSActive/1  "<VHAL_ABSActive_flg>"
  True_VHAL_ABSActive_flg/1 -> ABSActive/2
  [inp_CanValid_bus] -> slr1_3/1
  slr1_3/1 -> ABSActive/3  "<VINP_CANMsgValidESC1_flg>"
  ABSActive/1 -> VINP_ABSActive_flg/1  "VINP_ABSActive_flg"
  ABSActive/2 -> Terminator_3/1
  [BHAL_outputs] -> slr_VHAL_ABSFailed_flg/1
  slr_VHAL_ABSFailed_flg/1 -> ABSFailed/1  "<VHAL_ABSFailed_flg>"
  True_VHAL_ABSFailed_flg/1 -> ABSFailed/2
  [inp_CanValid_bus] -> slr1_4/1
  slr1_4/1 -> ABSFailed/3  "<VINP_CANMsgValidESC1_flg>"
  ABSFailed/1 -> VINP_ABSFailed_flg/1  "VINP_ABSFailed_flg"
  ABSFailed/2 -> Terminator_4/1
  [BHAL_outputs] -> slr_VHAL_ABSWnlmpSta_flg/1
  slr_VHAL_ABSWnlmpSta_flg/1 -> ABSWnlmpSta/1  "<VHAL_ABSWnlmpSta_flg>"
  True_VHAL_ABSWnlmpSta_flg/1 -> ABSWnlmpSta/2
  [inp_CanValid_bus] -> slr1_5/1
  slr1_5/1 -> ABSWnlmpSta/3  "<VINP_CANMsgValidESC1_flg>"
  ABSWnlmpSta/1 -> VINP_ABSWnlmpSta_flg/1  "VINP_ABSWnlmpSta_flg"
  ABSWnlmpSta/2 -> Terminator_5/1
  [BHAL_outputs] -> slr_VHAL_AVHActive_flg/1
  slr_VHAL_AVHActive_flg/1 -> AVHActive/1  "<VHAL_AVHActive_flg>"
  True_VHAL_AVHActive_flg/1 -> AVHActive/2
  [inp_CanValid_bus] -> slr1_6/1
  slr1_6/1 -> AVHActive/3  "<VINP_CANMsgValidESC1_flg>"
  AVHActive/1 -> VINP_AVHActive_flg/1  "VINP_AVHActive_flg"
  AVHActive/2 -> Terminator_6/1
  [BHAL_outputs] -> slr_VHAL_AVHFailed_flg/1
  slr_VHAL_AVHFailed_flg/1 -> AVHFailed/1  "<VHAL_AVHFailed_flg>"
  True_VHAL_AVHFailed_flg/1 -> AVHFailed/2
  [inp_CanValid_bus] -> slr1_7/1
  slr1_7/1 -> AVHFailed/3  "<VINP_CANMsgValidESC1_flg>"
  AVHFailed/1 -> VINP_AVHFailed_flg/1  "VINP_AVHFailed_flg"
  AVHFailed/2 -> Terminator_7/1
  [BHAL_outputs] -> slr_VHAL_AmberWnlmpSta_flg/1
  slr_VHAL_AmberWnlmpSta_flg/1 -> AmberWnlmpSta/1  "<VHAL_AmberWnlmpSta_flg>"
  True_VHAL_AmberWnlmpSta_flg/1 -> AmberWnlmpSta/2
  [inp_CanValid_bus] -> slr1_8/1
  slr1_8/1 -> AmberWnlmpSta/3  "<VINP_CANMsgValidESC1_flg>"
  AmberWnlmpSta/1 -> VINP_AmberWnlmpSta_flg/1  "VINP_AmberWnlmpSta_flg"
  AmberWnlmpSta/2 -> Terminator_8/1
  [BHAL_outputs] -> slr_VHAL_BTCSActive_flg/1
  slr_VHAL_BTCSActive_flg/1 -> BTCSActive/1  "<VHAL_BTCSActive_flg>"
  True_VHAL_BTCSActive_flg/1 -> BTCSActive/2
  [inp_CanValid_bus] -> slr1_9/1
  slr1_9/1 -> BTCSActive/3  "<VINP_CANMsgValidESC1_flg>"
  BTCSActive/1 -> VINP_BTCSActive_flg/1  "VINP_BTCSActive_flg"
  BTCSActive/2 -> Terminator_9/1
  [BHAL_outputs] -> slr_VHAL_EBDActive_flg/1
  slr_VHAL_EBDActive_flg/1 -> EBDActive/1  "<VHAL_EBDActive_flg>"
  True_VHAL_EBDActive_flg/1 -> EBDActive/2
  [inp_CanValid_bus] -> slr1_10/1
  slr1_10/1 -> EBDActive/3  "<VINP_CANMsgValidESC1_flg>"
  EBDActive/1 -> VINP_EBDActive_flg/1  "VINP_EBDActive_flg"
  EBDActive/2 -> Terminator_10/1
  [BHAL_outputs] -> slr_VHAL_EBDFailed_flg/1
  slr_VHAL_EBDFailed_flg/1 -> EBDFailed/1  "<VHAL_EBDFailed_flg>"
  True_VHAL_EBDFailed_flg/1 -> EBDFailed/2
  [inp_CanValid_bus] -> slr1_11/1
  slr1_11/1 -> EBDFailed/3  "<VINP_CANMsgValidESC1_flg>"
  EBDFailed/1 -> VINP_EBDFailed_flg/1  "VINP_EBDFailed_flg"
  EBDFailed/2 -> Terminator_11/1
  [BHAL_outputs] -> slr_VHAL_ESC1CS_enum/1
  slr_VHAL_ESC1CS_enum/1 -> ESC1CS/1  "<VHAL_ESC1CS_enum>"
  True_VHAL_ESC1CS_enum/1 -> ESC1CS/2
  [inp_CanValid_bus] -> slr1_12/1
  slr1_12/1 -> ESC1CS/3  "<VINP_CANMsgValidESC1_flg>"
  ESC1CS/1 -> VINP_ESC1CS_enum/1  "VINP_ESC1CS_enum"
  ESC1CS/2 -> Terminator_12/1
  [BHAL_outputs] -> slr_VHAL_ESC1RC_enum/1
  slr_VHAL_ESC1RC_enum/1 -> ESC1RC/1  "<VHAL_ESC1RC_enum>"
  True_VHAL_ESC1RC_enum/1 -> ESC1RC/2
  [inp_CanValid_bus] -> slr1_13/1
  slr1_13/1 -> ESC1RC/3  "<VINP_CANMsgValidESC1_flg>"
  ESC1RC/1 -> VINP_ESC1RC_enum/1  "VINP_ESC1RC_enum"
  ESC1RC/2 -> Terminator_13/1
  [BHAL_outputs] -> slr_VHAL_ESCActive_flg/1
  slr_VHAL_ESCActive_flg/1 -> ESCActive/1  "<VHAL_ESCActive_flg>"
  True_VHAL_ESCActive_flg/1 -> ESCActive/2
  [inp_CanValid_bus] -> slr1_14/1
  slr1_14/1 -> ESCActive/3  "<VINP_CANMsgValidESC1_flg>"
  ESCActive/1 -> VINP_ESCActive_flg/1  "VINP_ESCActive_flg"
  ESCActive/2 -> Terminator_14/1
  [BHAL_outputs] -> slr_VHAL_ESCBeepReq_flg/1
  slr_VHAL_ESCBeepReq_flg/1 -> ESCBeepReq/1  "<VHAL_ESCBeepReq_flg>"
  True_VHAL_ESCBeepReq_flg/1 -> ESCBeepReq/2
  [inp_CanValid_bus] -> slr1_15/1
  slr1_15/1 -> ESCBeepReq/3  "<VINP_CANMsgValidESC1_flg>"
  ESCBeepReq/1 -> VINP_ESCBeepReq_flg/1  "VINP_ESCBeepReq_flg"
  ESCBeepReq/2 -> Terminator_15/1
  [BHAL_outputs] -> slr_VHAL_ESCFailed_flg/1
  slr_VHAL_ESCFailed_flg/1 -> ESCFailed/1  "<VHAL_ESCFailed_flg>"
  True_VHAL_ESCFailed_flg/1 -> ESCFailed/2
  [inp_CanValid_bus] -> slr1_16/1
  slr1_16/1 -> ESCFailed/3  "<VINP_CANMsgValidESC1_flg>"
  ESCFailed/1 -> VINP_ESCFailed_flg/1  "VINP_ESCFailed_flg"
  ESCFailed/2 -> Terminator_16/1
  [BHAL_outputs] -> slr_VHAL_ESCOFFStatus_enum/1
  slr_VHAL_ESCOFFStatus_enum/1 -> ESCOFFStatus/1  "<VHAL_ESCOFFStatus_enum>"
  True_VHAL_ESCOFFStatus_enum/1 -> ESCOFFStatus/2
  [inp_CanValid_bus] -> slr1_17/1
  slr1_17/1 -> ESCOFFStatus/3  "<VINP_CANMsgValidESC1_flg>"
  ESCOFFStatus/1 -> VINP_ESCOFFStatus_enum/1  "VINP_ESCOFFStatus_enum"
  ESCOFFStatus/2 -> Terminator_17/1
  [BHAL_outputs] -> slr_VHAL_ESCOfflmpSta_flg/1
  slr_VHAL_ESCOfflmpSta_flg/1 -> ESCOfflmpSta/1  "<VHAL_ESCOfflmpSta_flg>"
  True_VHAL_ESCOfflmpSta_flg/1 -> ESCOfflmpSta/2
  [inp_CanValid_bus] -> slr1_18/1
  slr1_18/1 -> ESCOfflmpSta/3  "<VINP_CANMsgValidESC1_flg>"
  ESCOfflmpSta/1 -> VINP_ESCOfflmpSta_flg/1  "VINP_ESCOfflmpSta_flg"
  ESCOfflmpSta/2 -> Terminator_18/1
  [BHAL_outputs] -> slr_VHAL_ESCWnlmpSta_enum/1
  slr_VHAL_ESCWnlmpSta_enum/1 -> ESCWnlmpSta/1  "<VHAL_ESCWnlmpSta_enum>"
  True_VHAL_ESCWnlmpSta_enum/1 -> ESCWnlmpSta/2
  [inp_CanValid_bus] -> slr1_19/1
  slr1_19/1 -> ESCWnlmpSta/3  "<VINP_CANMsgValidESC1_flg>"
  ESCWnlmpSta/1 -> VINP_ESCWnlmpSta_enum/1  "VINP_ESCWnlmpSta_enum"
  ESCWnlmpSta/2 -> Terminator_19/1
  [BHAL_outputs] -> slr_VHAL_ESSActive_flg/1
  slr_VHAL_ESSActive_flg/1 -> ESSActive/1  "<VHAL_ESSActive_flg>"
  True_VHAL_ESSActive_flg/1 -> ESSActive/2
  [inp_CanValid_bus] -> slr1_20/1
  slr1_20/1 -> ESSActive/3  "<VINP_CANMsgValidESC1_flg>"
  ESSActive/1 -> VINP_ESSActive_flg/1  "VINP_ESSActive_flg"
  ESSActive/2 -> Terminator_20/1
  [BHAL_outputs] -> slr_VHAL_FrPTCSActive_flg/1
  slr_VHAL_FrPTCSActive_flg/1 -> FrPTCSActive/1  "<VHAL_FrPTCSActive_flg>"
  True_VHAL_FrPTCSActive_flg/1 -> FrPTCSActive/2
  [inp_CanValid_bus] -> slr1_21/1
  slr1_21/1 -> FrPTCSActive/3  "<VINP_CANMsgValidESC1_flg>"
  FrPTCSActive/1 -> VINP_FrPTCSActive_flg/1  "VINP_FrPTCSActive_flg"
  FrPTCSActive/2 -> Terminator_21/1
  [BHAL_outputs] -> slr_VHAL_FrntAxlTrqReqDrv_Nm/1
  slr_VHAL_FrntAxlTrqReqDrv_Nm/1 -> FrntAxlTrqReqDrv/1  "<VHAL_FrntAxlTrqReqDrv_Nm>"
  True_VHAL_FrntAxlTrqReqDrv_Nm/1 -> FrntAxlTrqReqDrv/2
  [inp_CanValid_bus] -> slr1_22/1
  slr1_22/1 -> FrntAxlTrqReqDrv/3  "<VINP_CANMsgValidESC1_flg>"
  FrntAxlTrqReqDrv/1 -> VINP_FrntAxlTrqReqDrv_Nm/1  "VINP_FrntAxlTrqReqDrv_Nm"
  FrntAxlTrqReqDrv/2 -> Terminator_22/1
  [BHAL_outputs] -> slr_VHAL_GRADE_Deg/1
  slr_VHAL_GRADE_Deg/1 -> GRADE/1  "<VHAL_GRADE_Deg>"
  True_VHAL_GRADE_Deg/1 -> GRADE/2
  [inp_CanValid_bus] -> slr1_23/1
  slr1_23/1 -> GRADE/3  "<VINP_CANMsgValidESC1_flg>"
  GRADE/1 -> VINP_GRADE_Deg/1  "VINP_GRADE_Deg"
  GRADE/2 -> Terminator_23/1
  [BHAL_outputs] -> slr_VHAL_HBBActive_flg/1
  slr_VHAL_HBBActive_flg/1 -> HBBActive/1  "<VHAL_HBBActive_flg>"
  True_VHAL_HBBActive_flg/1 -> HBBActive/2
  [inp_CanValid_bus] -> slr1_24/1
  slr1_24/1 -> HBBActive/3  "<VINP_CANMsgValidESC1_flg>"
  HBBActive/1 -> VINP_HBBActive_flg/1  "VINP_HBBActive_flg"
  HBBActive/2 -> Terminator_24/1
  [BHAL_outputs] -> slr_VHAL_HBBFailed_flg/1
  slr_VHAL_HBBFailed_flg/1 -> HBBFailed/1  "<VHAL_HBBFailed_flg>"
  True_VHAL_HBBFailed_flg/1 -> HBBFailed/2
  [inp_CanValid_bus] -> slr1_25/1
  slr1_25/1 -> HBBFailed/3  "<VINP_CANMsgValidESC1_flg>"
  HBBFailed/1 -> VINP_HBBFailed_flg/1  "VINP_HBBFailed_flg"
  HBBFailed/2 -> Terminator_25/1
  [BHAL_outputs] -> slr_VHAL_HDDActive_flg/1
  slr_VHAL_HDDActive_flg/1 -> HDDActive/1  "<VHAL_HDDActive_flg>"
  True_VHAL_HDDActive_flg/1 -> HDDActive/2
  [inp_CanValid_bus] -> slr1_26/1
  slr1_26/1 -> HDDActive/3  "<VINP_CANMsgValidESC1_flg>"
  HDDActive/1 -> VINP_HDDActive_flg/1  "VINP_HDDActive_flg"
  HDDActive/2 -> Terminator_26/1
  [BHAL_outputs] -> slr_VHAL_HDDFailed_flg/1
  slr_VHAL_HDDFailed_flg/1 -> HDDFailed/1  "<VHAL_HDDFailed_flg>"
  True_VHAL_HDDFailed_flg/1 -> HDDFailed/2
  [inp_CanValid_bus] -> slr1_27/1
  slr1_27/1 -> HDDFailed/3  "<VINP_CANMsgValidESC1_flg>"
  HDDFailed/1 -> VINP_HDDFailed_flg/1  "VINP_HDDFailed_flg"
  HDDFailed/2 -> Terminator_27/1
  [BHAL_outputs] -> slr_VHAL_HSAActive_flg/1
  slr_VHAL_HSAActive_flg/1 -> HSAActive/1  "<VHAL_HSAActive_flg>"
  True_VHAL_HSAActive_flg/1 -> HSAActive/2
  [inp_CanValid_bus] -> slr1_28/1
  slr1_28/1 -> HSAActive/3  "<VINP_CANMsgValidESC1_flg>"
  HSAActive/1 -> VINP_HSAActive_flg/1  "VINP_HSAActive_flg"
  HSAActive/2 -> Terminator_28/1
  [BHAL_outputs] -> slr_VHAL_HSAFailed_flg/1
  slr_VHAL_HSAFailed_flg/1 -> HSAFailed/1  "<VHAL_HSAFailed_flg>"
  True_VHAL_HSAFailed_flg/1 -> HSAFailed/2
  [inp_CanValid_bus] -> slr1_29/1
  slr1_29/1 -> HSAFailed/3  "<VINP_CANMsgValidESC1_flg>"
  HSAFailed/1 -> VINP_HSAFailed_flg/1  "VINP_HSAFailed_flg"
  HSAFailed/2 -> Terminator_29/1
  [BHAL_outputs] -> slr_VHAL_LFPulseCount_enum/1
  slr_VHAL_LFPulseCount_enum/1 -> LFPulseCount/1  "<VHAL_LFPulseCount_enum>"
  True_VHAL_LFPulseCount_enum/1 -> LFPulseCount/2
  [inp_CanValid_bus] -> slr1_30/1
  slr1_30/1 -> LFPulseCount/3  "<VINP_CANMsgValidESC1_flg>"
  LFPulseCount/1 -> VINP_LFPulseCount_enum/1  "VINP_LFPulseCount_enum"
  LFPulseCount/2 -> Terminator_30/1
  [BHAL_outputs] -> slr_VHAL_LFPulseCountV_flg/1
  slr_VHAL_LFPulseCountV_flg/1 -> LFPulseCountV/1  "<VHAL_LFPulseCountV_flg>"
  True_VHAL_LFPulseCountV_flg/1 -> LFPulseCountV/2
  [inp_CanValid_bus] -> slr1_31/1
  slr1_31/1 -> LFPulseCountV/3  "<VINP_CANMsgValidESC1_flg>"
  LFPulseCountV/1 -> VINP_LFPulseCountV_flg/1  "VINP_LFPulseCountV_flg"
  LFPulseCountV/2 -> Terminator_31/1
  [BHAL_outputs] -> slr_VHAL_LFRawWhlSpeed_kph/1
  slr_VHAL_LFRawWhlSpeed_kph/1 -> LFRawWhlSpeed/1  "<VHAL_LFRawWhlSpeed_kph>"
  True_VHAL_LFRawWhlSpeed_kph/1 -> LFRawWhlSpeed/2
  [inp_CanValid_bus] -> slr1_32/1
  slr1_32/1 -> LFRawWhlSpeed/3  "<VINP_CANMsgValidESC1_flg>"
  LFRawWhlSpeed/1 -> VINP_LFRawWhlSpeed_kph/1  "VINP_LFRawWhlSpeed_kph"
  LFRawWhlSpeed/2 -> Terminator_32/1
  [BHAL_outputs] -> slr_VHAL_LFRawWhlSpeedV_flg/1
  slr_VHAL_LFRawWhlSpeedV_flg/1 -> LFRawWhlSpeedV/1  "<VHAL_LFRawWhlSpeedV_flg>"
  True_VHAL_LFRawWhlSpeedV_flg/1 -> LFRawWhlSpeedV/2
  [inp_CanValid_bus] -> slr1_33/1
  slr1_33/1 -> LFRawWhlSpeedV/3  "<VINP_CANMsgValidESC1_flg>"
  LFRawWhlSpeedV/1 -> VINP_LFRawWhlSpeedV_flg/1  "VINP_LFRawWhlSpeedV_flg"
  LFRawWhlSpeedV/2 -> Terminator_33/1
  [BHAL_outputs] -> slr_VHAL_LFWhlRotDir_enum/1
  slr_VHAL_LFWhlRotDir_enum/1 -> LFWhlRotDir/1  "<VHAL_LFWhlRotDir_enum>"
  True_VHAL_LFWhlRotDir_enum/1 -> LFWhlRotDir/2
  [inp_CanValid_bus] -> slr1_34/1
  slr1_34/1 -> LFWhlRotDir/3  "<VINP_CANMsgValidESC1_flg>"
  LFWhlRotDir/1 -> VINP_LFWhlRotDir_enum/1  "VINP_LFWhlRotDir_enum"
  LFWhlRotDir/2 -> Terminator_34/1
  [BHAL_outputs] -> slr_VHAL_LRPulseCount_enum/1
  slr_VHAL_LRPulseCount_enum/1 -> LRPulseCount/1  "<VHAL_LRPulseCount_enum>"
  True_VHAL_LRPulseCount_enum/1 -> LRPulseCount/2
  [inp_CanValid_bus] -> slr1_35/1
  slr1_35/1 -> LRPulseCount/3  "<VINP_CANMsgValidESC1_flg>"
  LRPulseCount/1 -> VINP_LRPulseCount_enum/1  "VINP_LRPulseCount_enum"
  LRPulseCount/2 -> Terminator_35/1
  [BHAL_outputs] -> slr_VHAL_LRPulseCountV_flg/1
  slr_VHAL_LRPulseCountV_flg/1 -> LRPulseCountV/1  "<VHAL_LRPulseCountV_flg>"
  True_VHAL_LRPulseCountV_flg/1 -> LRPulseCountV/2
  [inp_CanValid_bus] -> slr1_36/1
  slr1_36/1 -> LRPulseCountV/3  "<VINP_CANMsgValidESC1_flg>"
  LRPulseCountV/1 -> VINP_LRPulseCountV_flg/1  "VINP_LRPulseCountV_flg"
  LRPulseCountV/2 -> Terminator_36/1
  [BHAL_outputs] -> slr_VHAL_LRRawWhlSpeed_kph/1
  slr_VHAL_LRRawWhlSpeed_kph/1 -> LRRawWhlSpeed/1  "<VHAL_LRRawWhlSpeed_kph>"
  True_VHAL_LRRawWhlSpeed_kph/1 -> LRRawWhlSpeed/2
  [inp_CanValid_bus] -> slr1_37/1
  slr1_37/1 -> LRRawWhlSpeed/3  "<VINP_CANMsgValidESC1_flg>"
  LRRawWhlSpeed/1 -> VINP_LRRawWhlSpeed_kph/1  "VINP_LRRawWhlSpeed_kph"
  LRRawWhlSpeed/2 -> Terminator_37/1
  [BHAL_outputs] -> slr_VHAL_LRRawWhlSpeedV_flg/1
  slr_VHAL_LRRawWhlSpeedV_flg/1 -> LRRawWhlSpeedV/1  "<VHAL_LRRawWhlSpeedV_flg>"
  True_VHAL_LRRawWhlSpeedV_flg/1 -> LRRawWhlSpeedV/2
  [inp_CanValid_bus] -> slr1_38/1
  slr1_38/1 -> LRRawWhlSpeedV/3  "<VINP_CANMsgValidESC1_flg>"
  LRRawWhlSpeedV/1 -> VINP_LRRawWhlSpeedV_flg/1  "VINP_LRRawWhlSpeedV_flg"
  LRRawWhlSpeedV/2 -> Terminator_38/1
  [BHAL_outputs] -> slr_VHAL_LRWhlRotDir_enum/1
  slr_VHAL_LRWhlRotDir_enum/1 -> LRWhlRotDir/1  "<VHAL_LRWhlRotDir_enum>"
  True_VHAL_LRWhlRotDir_enum/1 -> LRWhlRotDir/2
  [inp_CanValid_bus] -> slr1_39/1
  slr1_39/1 -> LRWhlRotDir/3  "<VINP_CANMsgValidESC1_flg>"
  LRWhlRotDir/1 -> VINP_LRWhlRotDir_enum/1  "VINP_LRWhlRotDir_enum"
  LRWhlRotDir/2 -> Terminator_39/1
  [BHAL_outputs] -> slr_VHAL_PBAActive_flg/1
  slr_VHAL_PBAActive_flg/1 -> PBAActive/1  "<VHAL_PBAActive_flg>"
  True_VHAL_PBAActive_flg/1 -> PBAActive/2
  [inp_CanValid_bus] -> slr1_40/1
  slr1_40/1 -> PBAActive/3  "<VINP_CANMsgValidESC1_flg>"
  PBAActive/1 -> VINP_PBAActive_flg/1  "VINP_PBAActive_flg"
  PBAActive/2 -> Terminator_40/1
  [BHAL_outputs] -> slr_VHAL_PBAFailed_flg/1
  slr_VHAL_PBAFailed_flg/1 -> PBAFailed/1  "<VHAL_PBAFailed_flg>"
  True_VHAL_PBAFailed_flg/1 -> PBAFailed/2
  [inp_CanValid_bus] -> slr1_41/1
  slr1_41/1 -> PBAFailed/3  "<VINP_CANMsgValidESC1_flg>"
  PBAFailed/1 -> VINP_PBAFailed_flg/1  "VINP_PBAFailed_flg"
  PBAFailed/2 -> Terminator_41/1
  [BHAL_outputs] -> slr_VHAL_RFPulseCount_enum/1
  slr_VHAL_RFPulseCount_enum/1 -> RFPulseCount/1  "<VHAL_RFPulseCount_enum>"
  True_VHAL_RFPulseCount_enum/1 -> RFPulseCount/2
  [inp_CanValid_bus] -> slr1_42/1
  slr1_42/1 -> RFPulseCount/3  "<VINP_CANMsgValidESC1_flg>"
  RFPulseCount/1 -> VINP_RFPulseCount_enum/1  "VINP_RFPulseCount_enum"
  RFPulseCount/2 -> Terminator_42/1
  [BHAL_outputs] -> slr_VHAL_RFPulseCountV_flg/1
  slr_VHAL_RFPulseCountV_flg/1 -> RFPulseCountV/1  "<VHAL_RFPulseCountV_flg>"
  True_VHAL_RFPulseCountV_flg/1 -> RFPulseCountV/2
  [inp_CanValid_bus] -> slr1_43/1
  slr1_43/1 -> RFPulseCountV/3  "<VINP_CANMsgValidESC1_flg>"
  RFPulseCountV/1 -> VINP_RFPulseCountV_flg/1  "VINP_RFPulseCountV_flg"
  RFPulseCountV/2 -> Terminator_43/1
  [BHAL_outputs] -> slr_VHAL_RFRawWhlSpeed_kph/1
  slr_VHAL_RFRawWhlSpeed_kph/1 -> RFRawWhlSpeed/1  "<VHAL_RFRawWhlSpeed_kph>"
  True_VHAL_RFRawWhlSpeed_kph/1 -> RFRawWhlSpeed/2
  [inp_CanValid_bus] -> slr1_44/1
  slr1_44/1 -> RFRawWhlSpeed/3  "<VINP_CANMsgValidESC1_flg>"
  RFRawWhlSpeed/1 -> VINP_RFRawWhlSpeed_kph/1  "VINP_RFRawWhlSpeed_kph"
  RFRawWhlSpeed/2 -> Terminator_44/1
  [BHAL_outputs] -> slr_VHAL_RFRawWhlSpeedV_flg/1
  slr_VHAL_RFRawWhlSpeedV_flg/1 -> RFRawWhlSpeedV/1  "<VHAL_RFRawWhlSpeedV_flg>"
  True_VHAL_RFRawWhlSpeedV_flg/1 -> RFRawWhlSpeedV/2
  [inp_CanValid_bus] -> slr1_45/1
  slr1_45/1 -> RFRawWhlSpeedV/3  "<VINP_CANMsgValidESC1_flg>"
  RFRawWhlSpeedV/1 -> VINP_RFRawWhlSpeedV_flg/1  "VINP_RFRawWhlSpeedV_flg"
  RFRawWhlSpeedV/2 -> Terminator_45/1
  [BHAL_outputs] -> slr_VHAL_RFWhlRotDir_enum/1
  slr_VHAL_RFWhlRotDir_enum/1 -> RFWhlRotDir/1  "<VHAL_RFWhlRotDir_enum>"
  True_VHAL_RFWhlRotDir_enum/1 -> RFWhlRotDir/2
  [inp_CanValid_bus] -> slr1_46/1
  slr1_46/1 -> RFWhlRotDir/3  "<VINP_CANMsgValidESC1_flg>"
  RFWhlRotDir/1 -> VINP_RFWhlRotDir_enum/1  "VINP_RFWhlRotDir_enum"
  RFWhlRotDir/2 -> Terminator_46/1
  [BHAL_outputs] -> slr_VHAL_RRPulseCount_enum/1
  slr_VHAL_RRPulseCount_enum/1 -> RRPulseCount/1  "<VHAL_RRPulseCount_enum>"
  True_VHAL_RRPulseCount_enum/1 -> RRPulseCount/2
  [inp_CanValid_bus] -> slr1_47/1
  slr1_47/1 -> RRPulseCount/3  "<VINP_CANMsgValidESC1_flg>"
  RRPulseCount/1 -> VINP_RRPulseCount_enum/1  "VINP_RRPulseCount_enum"
  RRPulseCount/2 -> Terminator_47/1
  [BHAL_outputs] -> slr_VHAL_RRPulseCountV_flg/1
  slr_VHAL_RRPulseCountV_flg/1 -> RRPulseCountV/1  "<VHAL_RRPulseCountV_flg>"
  True_VHAL_RRPulseCountV_flg/1 -> RRPulseCountV/2
  [inp_CanValid_bus] -> slr1_48/1
  slr1_48/1 -> RRPulseCountV/3  "<VINP_CANMsgValidESC1_flg>"
  RRPulseCountV/1 -> VINP_RRPulseCountV_flg/1  "VINP_RRPulseCountV_flg"
  RRPulseCountV/2 -> Terminator_48/1
  [BHAL_outputs] -> slr_VHAL_RRRawWhlSpeed_kph/1
  slr_VHAL_RRRawWhlSpeed_kph/1 -> RRRawWhlSpeed/1  "<VHAL_RRRawWhlSpeed_kph>"
  True_VHAL_RRRawWhlSpeed_kph/1 -> RRRawWhlSpeed/2
  [inp_CanValid_bus] -> slr1_49/1
  slr1_49/1 -> RRRawWhlSpeed/3  "<VINP_CANMsgValidESC1_flg>"
  RRRawWhlSpeed/1 -> VINP_RRRawWhlSpeed_kph/1  "VINP_RRRawWhlSpeed_kph"
  RRRawWhlSpeed/2 -> Terminator_49/1
  [BHAL_outputs] -> slr_VHAL_RRRawWhlSpeedV_flg/1
  slr_VHAL_RRRawWhlSpeedV_flg/1 -> RRRawWhlSpeedV/1  "<VHAL_RRRawWhlSpeedV_flg>"
  True_VHAL_RRRawWhlSpeedV_flg/1 -> RRRawWhlSpeedV/2
  [inp_CanValid_bus] -> slr1_50/1
  slr1_50/1 -> RRRawWhlSpeedV/3  "<VINP_CANMsgValidESC1_flg>"
  RRRawWhlSpeedV/1 -> VINP_RRRawWhlSpeedV_flg/1  "VINP_RRRawWhlSpeedV_flg"
  RRRawWhlSpeedV/2 -> Terminator_50/1
  [BHAL_outputs] -> slr_VHAL_RRWhlRotDir_enum/1
  slr_VHAL_RRWhlRotDir_enum/1 -> RRWhlRotDir/1  "<VHAL_RRWhlRotDir_enum>"
  True_VHAL_RRWhlRotDir_enum/1 -> RRWhlRotDir/2
  [inp_CanValid_bus] -> slr1_51/1
  slr1_51/1 -> RRWhlRotDir/3  "<VINP_CANMsgValidESC1_flg>"
  RRWhlRotDir/1 -> VINP_RRWhlRotDir_enum/1  "VINP_RRWhlRotDir_enum"
  RRWhlRotDir/2 -> Terminator_51/1
  [BHAL_outputs] -> slr_VHAL_RearAxlTrqReqDrv_Nm/1
  slr_VHAL_RearAxlTrqReqDrv_Nm/1 -> RearAxlTrqReqDrv/1  "<VHAL_RearAxlTrqReqDrv_Nm>"
  True_VHAL_RearAxlTrqReqDrv_Nm/1 -> RearAxlTrqReqDrv/2
  [inp_CanValid_bus] -> slr1_52/1
  slr1_52/1 -> RearAxlTrqReqDrv/3  "<VINP_CANMsgValidESC1_flg>"
  RearAxlTrqReqDrv/1 -> VINP_RearAxlTrqReqDrv_Nm/1  "VINP_RearAxlTrqReqDrv_Nm"
  RearAxlTrqReqDrv/2 -> Terminator_52/1
  [BHAL_outputs] -> slr_VHAL_RedWnlmpSta_flg/1
  slr_VHAL_RedWnlmpSta_flg/1 -> RedWnlmpSta/1  "<VHAL_RedWnlmpSta_flg>"
  True_VHAL_RedWnlmpSta_flg/1 -> RedWnlmpSta/2
  [inp_CanValid_bus] -> slr1_53/1
  slr1_53/1 -> RedWnlmpSta/3  "<VINP_CANMsgValidESC1_flg>"
  RedWnlmpSta/1 -> VINP_RedWnlmpSta_flg/1  "VINP_RedWnlmpSta_flg"
  RedWnlmpSta/2 -> Terminator_53/1
  [BHAL_outputs] -> slr_VHAL_RrPTCSActive_flg/1
  slr_VHAL_RrPTCSActive_flg/1 -> RrPTCSActive/1  "<VHAL_RrPTCSActive_flg>"
  True_VHAL_RrPTCSActive_flg/1 -> RrPTCSActive/2
  [inp_CanValid_bus] -> slr1_54/1
  slr1_54/1 -> RrPTCSActive/3  "<VINP_CANMsgValidESC1_flg>"
  RrPTCSActive/1 -> VINP_RrPTCSActive_flg/1  "VINP_RrPTCSActive_flg"
  RrPTCSActive/2 -> Terminator_54/1
  [BHAL_outputs] -> slr_VHAL_TCSActive_flg/1
  slr_VHAL_TCSActive_flg/1 -> TCSActive/1  "<VHAL_TCSActive_flg>"
  True_VHAL_TCSActive_flg/1 -> TCSActive/2
  [inp_CanValid_bus] -> slr1_55/1
  slr1_55/1 -> TCSActive/3  "<VINP_CANMsgValidESC1_flg>"
  TCSActive/1 -> VINP_TCSActive_flg/1  "VINP_TCSActive_flg"
  TCSActive/2 -> Terminator_55/1
  [BHAL_outputs] -> slr_VHAL_TCSFailed_flg/1
  slr_VHAL_TCSFailed_flg/1 -> TCSFailed/1  "<VHAL_TCSFailed_flg>"
  True_VHAL_TCSFailed_flg/1 -> TCSFailed/2
  [inp_CanValid_bus] -> slr1_56/1
  slr1_56/1 -> TCSFailed/3  "<VINP_CANMsgValidESC1_flg>"
  TCSFailed/1 -> VINP_TCSFailed_flg/1  "VINP_TCSFailed_flg"
  TCSFailed/2 -> Terminator_56/1
  [BHAL_outputs] -> slr_VHAL_VehSpeed_kph/1
  slr_VHAL_VehSpeed_kph/1 -> VehSpeed/1  "<VHAL_VehSpeed_kph>"
  True_VHAL_VehSpeed_kph/1 -> VehSpeed/2
  [inp_CanValid_bus] -> slr1_57/1
  slr1_57/1 -> VehSpeed/3  "<VINP_CANMsgValidESC1_flg>"
  VehSpeed/1 -> VINP_VehSpeed_kph/1  "VINP_VehSpeed_kph"
  VehSpeed/2 -> Terminator_57/1
